simulink library "photodiodes_lib"  (R2016b)
settings: Solver=VariableStepAuto  StartTime=0.0  StopTime=10.0  RelTol=1e-3
libraries: dspmathops x2
settings Model: Creator=Taylor  LastModifiedBy=Taylor

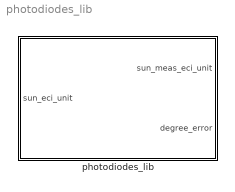
== system photodiodes_lib ==
  photodiodes_lib : Subsystem

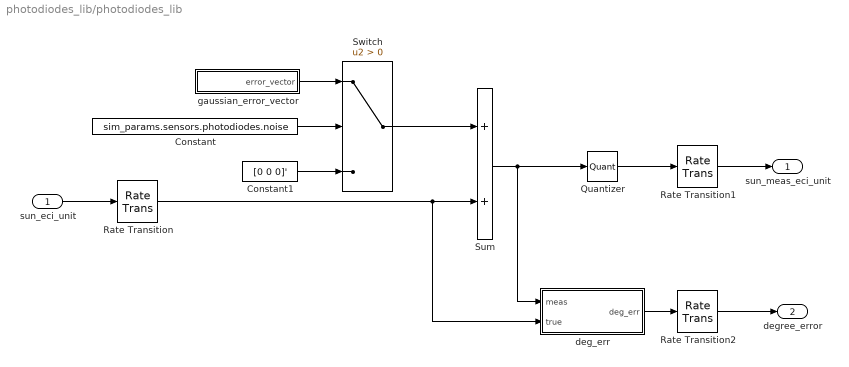
== system photodiodes_lib/photodiodes_lib ==
  sun_eci_unit : Inport
  Constant : Constant  Value=sim_params.sensors.photodiodes.noise  SampleTime=sim_params.sensors.photodiodes.sample_time_s
  Constant1 : Constant  Value=[0 0 0]'  SampleTime=sim_params.sensors.photodiodes.sample_time_s
  Quantizer : Quantizer  QuantizationInterval=sim_params.sensors.photodiodes.resolution
  Rate Transition : RateTransition  OutPortSampleTime=sim_params.sensors.photodiodes.sample_time_s
  Rate Transition1 : RateTransition
  Rate Transition2 : RateTransition
  Sum : Sum
  Switch : Switch  Criteria=u2 > Threshold
  deg_err : Subsystem
  gaussian_error_vector : Subsystem
  sun_meas_eci_unit : Outport
  "degree_error " : Outport  Port=2
  wires:
  Switch/1 -> Sum/1
  Constant1/1 -> Switch/3
  gaussian_error_vector/1(error_vector) -> Switch/1
  sun_eci_unit/1 -> Rate Transition/1
  deg_err/1(deg_err) -> Rate Transition2/1
  Sum/1 -> Quantizer/1, deg_err/1(meas)
  Constant/1 -> Switch/2
  Quantizer/1 -> Rate Transition1/1
  Rate Transition/1 -> deg_err/2(true), Sum/2
  Rate Transition1/1 -> sun_meas_eci_unit/1
  Rate Transition2/1 -> "degree_error "/1

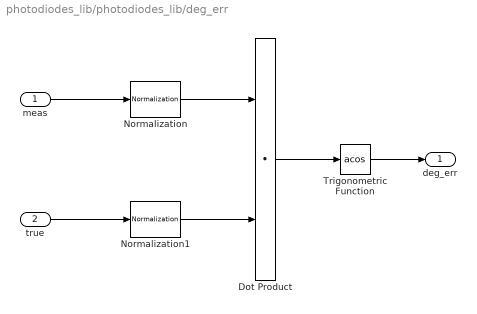
== system photodiodes_lib/photodiodes_lib/deg_err ==
  meas : Inport
  true : Inport  Port=2
  Dot Product : DotProduct  InputSameDT=on  OutDataTypeStr=Inherit: Inherit via internal rule
  Normalization : dspmathops/Normalization  NormType=2-norm  Bias=1e-10  NormOver=Each column  Dimension=1  outputDataTypeStr=Inherit: Same as product output  outputLastDataTypeStr=Inherit: Same as product output  outputMin=[]  outputMax=[]  accumDataTypeStr=Inherit: Same as product output  accumLastDataTypeStr=Inherit: Same as product output  roundingMode=Floor  overflowMode=off
  Normalization1 : dspmathops/Normalization  NormType=2-norm  Bias=1e-10  NormOver=Each column  Dimension=1  outputDataTypeStr=Inherit: Same as product output  outputLastDataTypeStr=Inherit: Same as product output  outputMin=[]  outputMax=[]  accumDataTypeStr=Inherit: Same as product output  accumLastDataTypeStr=Inherit: Same as product output  roundingMode=Floor  overflowMode=off
  Trigonometric Function : Trigonometry  Operator=acos
  deg_err : Outport
  wires:
  meas/1 -> Normalization/1
  Dot Product/1 -> Trigonometric Function/1
  Trigonometric Function/1 -> deg_err/1
  true/1 -> Normalization1/1
  Normalization/1 -> Dot Product/1
  Normalization1/1 -> Dot Product/2

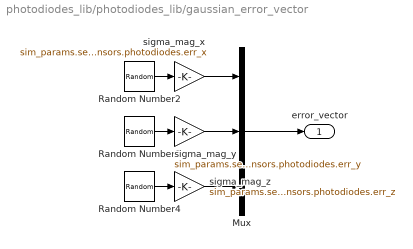
== system photodiodes_lib/photodiodes_lib/gaussian_error_vector ==
  Mux : Mux  Inputs=3
  Random Number2 : RandomNumber  SampleTime=sim_params.sensors.photodiodes.sample_time_s
  Random Number3 : RandomNumber  Seed=1  SampleTime=sim_params.sensors.photodiodes.sample_time_s
  Random Number4 : RandomNumber  Seed=2  SampleTime=sim_params.sensors.photodiodes.sample_time_s
  sigma_mag_x : Gain  Gain=sim_params.sensors.photodiodes.err_x
  sigma_mag_y : Gain  Gain=sim_params.sensors.photodiodes.err_y
  sigma_mag_z : Gain  Gain=sim_params.sensors.photodiodes.err_z
  error_vector : Outport
  wires:
  Random Number2/1 -> sigma_mag_x/1
  Random Number4/1 -> sigma_mag_z/1
  Random Number3/1 -> sigma_mag_y/1
  sigma_mag_x/1 -> Mux/1
  sigma_mag_y/1 -> Mux/2
  Mux/1 -> error_vector/1
  sigma_mag_z/1 -> Mux/3
